simulink model "seMM1QueuingSys"  (R2024a)
settings: Solver=VariableStepAuto  StartTime=0.0  StopTime=60  RelTol=1e-3  EnableMultiTasking=on
model workspace (MAT data in the model file):
  GGwp = 5
undefined symbols (not defined in the file): m, n
libraries: commrandsrc3 x8, spsMonostableLib x4, simulink x2
settings Model: SimulationMode=accelerator  Creator=The MathWorks, Inc.  LastModifiedBy=94410
settings SolverCC: AlgebraicLoopSolver=TrustRegion
settings DataIOCC: LimitDataPoints=on  SaveFormat=Array  ReturnWorkspaceOutputs=off
settings OptimizationCC: LifeSpan=inf
settings DebuggingCC: UnconnectedInputMsg=warning  UnconnectedOutputMsg=warning  UnconnectedLineMsg=warning  AllowSymbolicDim=off  SFUnexpectedBacktrackingDiag=warning  SFNoUnconditionalDefaultTransitionDiag=warning  SFExecutionAtInitializationDiag=none  ArithmeticOperatorsInVariantConditions=warning
settings ModelReferenceCC: EnableRefExpFcnMdlSchedulingChecks=on  PropagateSignalLabelsOutOfModel=off
settings SFSimCC: SimUseLocalCustomCode=off  CustomCodeUndefinedFunction=UseInterfaceOnly
settings RTWCC: RTWUseLocalCustomCode=off  GPUComputeCapability=3.5  DLArmComputeVersion=19.05
settings CodeAppCC: StateflowObjectComments=on
settings GRTTargetCC: TargetLangStandard=C89/C90 (ANSI)
settings ConfigComp: CovMetricSettings=dw  CovSaveCumulativeToWorkspaceVar=on  CovSaveSingleToWorkspaceVar=on  CovExternalEMLEnable=off  CovSFcnEnable=off

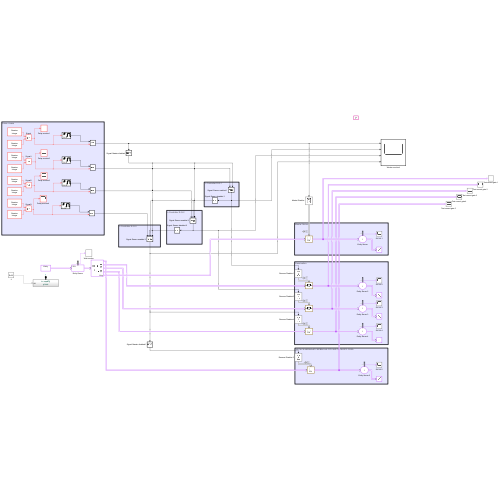
[thumbnail: Simulink's stored preview of the top-level diagram]
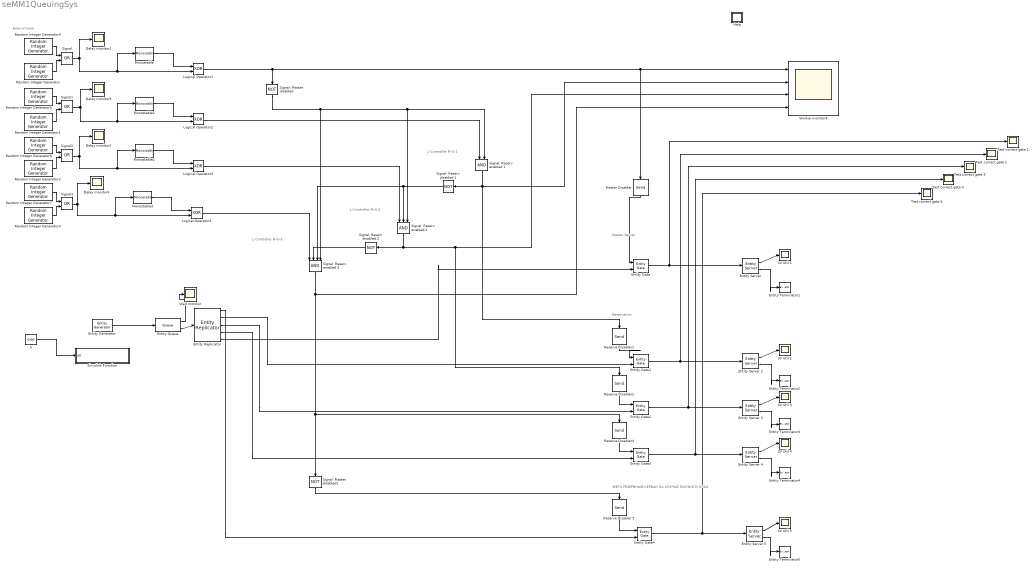
== system seMM1QueuingSys ==
  note: МЕГА РЕЗЕРВНЫЙ СЕРВАК НА СЛУЧАЙ ПОЛНОГО ОЧКА
  note: L-Controller R-G-3
  note: L-Controller R-G-2
  note: L-Controller R-G-1
  note: Reservation
  note: Master Server
  note: Блок отказа
  " λ" : Constant  Value=0.66  SampleTime=-1
  Delay monitor{1..4} (4 alike) : Scope
  Entity Gate{,1..4} (5 alike) : EntityGate  InputPortMessageModes=m,m  OutputPortMessageModes=m
  Entity Generator : EntityGenerator  OutputPortMessageModes=m  TimeSource=MATLAB action  Period=5  IntergenerationTimeAction=dt = expAT();  AttributeName=entity  AttributeInitialValue=0  EntityType=Structured  EntityTypeName=Entity
  Entity Queue : Queue  InputPortMessageModes=m  OutputPortMessageModes=n,m  Capacity=inf  AverageWait=on
      settings: OutputPortMap=o2,o5
  Entity Replicator : EntityReplicator  InputPortMessageModes=m  OutputPortMessageModes=m,m,m,m,m  NumberReplicas=4
      settings: OutputPortMap=o0,o1,o2,o3,o4
  Entity Server : EntityServer  InputPortMessageModes=m  OutputPortMessageModes=n,m  Capacity=1  ServiceTimeValue=2.0  Utilization=on
      settings: OutputPortMap=o5,o9
  Entity Server {2..5} (4 alike) : EntityServer  InputPortMessageModes=m  OutputPortMessageModes=n,m  Capacity=1  ServiceTimeValue=2.0  Utilization=on
      settings: OutputPortMap=o5,o9
  Entity Terminator{1..5} (5 alike) : EntityTerminator  InputPortMessageModes=m
  Help : Subsystem
      settings: OpenFcn=showExample('simevents/MM1QueuingSysExample');
      mask Display: disp('?')
  Logical Operator{1..4} (4 alike) : Logic  Operator=XOR  AllPortsSameDT=off  OutDataTypeStr=boolean
  Master Disabler : Send  OutputPortMessageModes=m
  Monostable{,1..3} (4 alike) : spsMonostableLib/Monostable  EdgeDetect=Rising  PulseDuration=0.5  ic=1  Ts=0
      settings: LibrarySourceBlock=sps_lib/Control/Monostable
  Random Integer Generator : commrandsrc3/Random Integer Generator  SetSize=2  SeedSource=Parameter  Seed=440  SampleTime=1  SamplesPerFrame=1  OutputDataType=boolean  SimulateUsing=Interpreted execution
  Random Integer Generator1 : commrandsrc3/Random Integer Generator  SetSize=2  SeedSource=Parameter  Seed=706  SampleTime=1  SamplesPerFrame=1  OutputDataType=boolean  SimulateUsing=Interpreted execution
  Random Integer Generator2 : commrandsrc3/Random Integer Generator  SetSize=2  SeedSource=Parameter  Seed=569  SampleTime=1  SamplesPerFrame=1  OutputDataType=boolean  SimulateUsing=Interpreted execution
  Random Integer Generator3 : commrandsrc3/Random Integer Generator  SetSize=2  SeedSource=Parameter  Seed=513  SampleTime=1  SamplesPerFrame=1  OutputDataType=boolean  SimulateUsing=Interpreted execution
  Random Integer Generator4 : commrandsrc3/Random Integer Generator  SetSize=2  SeedSource=Parameter  Seed=420  SampleTime=1  SamplesPerFrame=1  OutputDataType=boolean  SimulateUsing=Interpreted execution
  Random Integer Generator5 : commrandsrc3/Random Integer Generator  SetSize=2  SeedSource=Parameter  Seed=700  SampleTime=1  SamplesPerFrame=1  OutputDataType=boolean  SimulateUsing=Interpreted execution
  Random Integer Generator6 : commrandsrc3/Random Integer Generator  SetSize=2  SeedSource=Parameter  Seed=560  SampleTime=1  SamplesPerFrame=1  OutputDataType=boolean  SimulateUsing=Interpreted execution
  Random Integer Generator7 : commrandsrc3/Random Integer Generator  SetSize=2  SeedSource=Parameter  Seed=430  SampleTime=1  SamplesPerFrame=1  OutputDataType=boolean  SimulateUsing=Interpreted execution
  Reserve Disabler 5 : Send  OutputPortMessageModes=m
  Reserve Disabler1 : Send  OutputPortMessageModes=m
  Reserve Disabler2 : Send  OutputPortMessageModes=m
  Reserve Disabler4 : Send  OutputPortMessageModes=m
  SV Util {1..5} (5 alike) : Scope
  Signal{,1..3} (4 alike) : Logic  Operator=OR  AllPortsSameDT=off  OutDataTypeStr=boolean
  Signal: Master disabled : Logic  Operator=NOT  AllPortsSameDT=off  OutDataTypeStr=boolean
  Signal: Master disabled1 : Logic  Operator=NOT  AllPortsSameDT=off  OutDataTypeStr=boolean
  Signal: Reserv disabled 1 : Logic  Operator=NOT  AllPortsSameDT=off  OutDataTypeStr=boolean
  Signal: Reserv disabled 2 : Logic  Operator=NOT  AllPortsSameDT=off  OutDataTypeStr=boolean
  Signal: Reserv enabled 1 : Logic  AllPortsSameDT=off  OutDataTypeStr=boolean
  Signal: Reserv enabled 2 : Logic  Inputs=3  AllPortsSameDT=off  OutDataTypeStr=boolean
  Signal: Reserv enabled 3 : Logic  Inputs=4  AllPortsSameDT=off  OutDataTypeStr=boolean
  Simulink Function : Subsystem  TreatAsAtomicUnit=on
  Test correct gate {1..5} (5 alike) : Scope
  Wait monitor : Scope
  Worker monitor4 : Scope  NumInputPorts=4
  wires:
  " λ"/1 -> Simulink Function/1(AR)
  Entity Gate/1 -> Entity Server/1, Test correct gate 1/1
  Entity Generator/1 -> Entity Queue/1
  Entity Gate1/1 -> Entity Server 2/1, Test correct gate 2/1
  Entity Queue/2 -> Entity Replicator/1
  Entity Queue/1 -> Wait monitor/1
  Entity Replicator/1 -> Entity Gate4/2
  Entity Replicator/2 -> Entity Gate1/2
  Entity Server/2 -> Entity Terminator1/1
  Entity Server 2/2 -> Entity Terminator2/1
  Signal/1 -> Delay monitor1/1, Monostable/1, Logical Operator1/2
  Entity Server/1 -> SV Util 1/1
  Entity Server 2/1 -> SV Util 2/1
  Monostable/1 -> Logical Operator1/1
  Monostable1/1 -> Logical Operator2/1
  Signal1/1 -> Delay monitor3/1, Monostable1/1, Logical Operator2/2
  Entity Server 3/1 -> SV Util 3/1
  Entity Server 4/1 -> SV Util 4/1
  Entity Server 4/2 -> Entity Terminator4/1
  Entity Server 3/2 -> Entity Terminator3/1
  Entity Replicator/3 -> Entity Gate2/2
  Entity Replicator/4 -> Entity Gate3/2
  Entity Gate2/1 -> Entity Server 3/1, Test correct gate 3/1
  Entity Gate3/1 -> Entity Server 4/1, Test correct gate 4/1
  Master Disabler/1 -> Entity Gate/1
  Logical Operator1/1 -> Master Disabler/1, Worker monitor4/1, Signal: Master disabled/1
  Reserve Disabler1/1 -> Entity Gate1/1
  Reserve Disabler2/1 -> Entity Gate2/1
  Reserve Disabler4/1 -> Entity Gate3/1
  Signal: Master disabled/1 -> Signal: Reserv enabled 3/4, Signal: Reserv enabled 2/3, Signal: Reserv enabled 1/2
  Logical Operator2/1 -> Signal: Reserv enabled 1/1
  Signal: Reserv enabled 1/1 -> Worker monitor4/2, Signal: Reserv disabled 1/1, Reserve Disabler1/1
  Signal2/1 -> Monostable2/1, Logical Operator3/2, Delay monitor2/1
  Monostable2/1 -> Logical Operator3/1
  Signal3/1 -> Delay monitor4/1, Monostable3/1, Logical Operator4/2
  Monostable3/1 -> Logical Operator4/1
  Signal: Reserv disabled 1/1 -> Signal: Reserv enabled 3/3, Signal: Reserv enabled 2/2
  Logical Operator3/1 -> Signal: Reserv enabled 2/1
  Signal: Reserv enabled 2/1 -> Worker monitor4/3, Reserve Disabler2/1, Signal: Reserv disabled 2/1
  Signal: Reserv disabled 2/1 -> Signal: Reserv enabled 3/2
  Logical Operator4/1 -> Signal: Reserv enabled 3/1
  Signal: Reserv enabled 3/1 -> Worker monitor4/4, Signal: Master disabled1/1, Reserve Disabler4/1
  Entity Gate4/1 -> Entity Server 5/1, Test correct gate 5/1
  Entity Server 5/1 -> SV Util 5/1
  Entity Server 5/2 -> Entity Terminator5/1
  Signal: Master disabled1/1 -> Reserve Disabler 5/1
  Entity Replicator/5 -> Entity Gate/2
  Reserve Disabler 5/1 -> Entity Gate4/1
  Random Integer Generator4/1 -> Signal/1
  Random Integer Generator/1 -> Signal/2
  Random Integer Generator5/1 -> Signal1/1
  Random Integer Generator1/1 -> Signal1/2
  Random Integer Generator6/1 -> Signal2/1
  Random Integer Generator2/1 -> Signal2/2
  Random Integer Generator7/1 -> Signal3/1
  Random Integer Generator3/1 -> Signal3/2

== system seMM1QueuingSys/Help ==

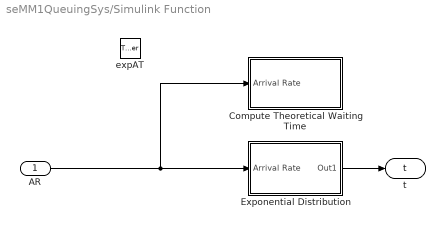
== system seMM1QueuingSys/Simulink Function ==
  AR : Inport
  expAT : TriggerPort  TriggerType=function-call  IsSimulinkFunction=on  FunctionName=expAT  VariantControl=Variant
  Compute Theoretical Waiting Time : Subsystem
  Exponential Distribution : Subsystem
  t : ArgOut  DisableCoverage=on  ArgumentName=t
  wires:
  AR/1 -> Compute Theoretical Waiting Time/1(Arrival Rate), Exponential Distribution/1(Arrival Rate)
  Exponential Distribution/1(Out1) -> t/1

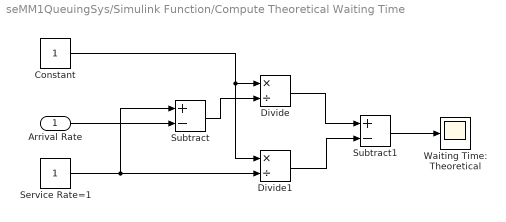
== system seMM1QueuingSys/Simulink Function/Compute Theoretical Waiting Time ==
  Arrival Rate : Inport
  Constant : Constant
  Divide : Product  Inputs=*/
  Divide1 : Product  Inputs=*/
  Service Rate=1 : Constant
  Subtract : Sum  Inputs=+-
  Subtract1 : Sum  Inputs=+-
  Waiting Time: Theoretical : Scope
  wires:
  Arrival Rate/1 -> Subtract/2
  Subtract1/1 -> Waiting Time: Theoretical/1
  Divide1/1 -> Subtract1/2
  Divide/1 -> Subtract1/1
  Subtract/1 -> Divide/2
  Constant/1 -> Divide1/1, Divide/1
  Service Rate=1/1 -> Subtract/1, Divide1/2

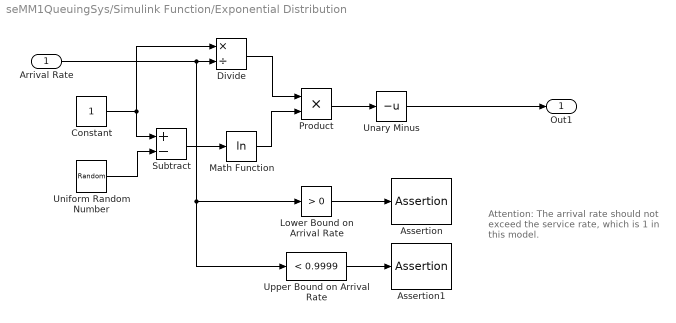
== system seMM1QueuingSys/Simulink Function/Exponential Distribution ==
  note: Attention: The arrival rate
      | should not exceed the service
      | rate, which is 1 in this model.
  Arrival Rate : Inport
  Assertion : Assertion
  Assertion1 : Assertion
  Constant : Constant
  Divide : Product  Inputs=*/
  Lower Bound on Arrival Rate : simulink/Logic and Bit Operations/Compare To Constant  relop=>  const=0  OutDataTypeStr=uint8  ZeroCross=off
  Math Function : Math  Operator=log  SignedPower=on
  Product : Product  RndMeth=Zero
  Subtract : Sum  Inputs=+-
  Unary Minus : UnaryMinus
  Uniform Random Number : UniformRandomNumber  Minimum=0  Seed=12345
  "Upper Bound on Arrival Rate " : simulink/Logic and Bit Operations/Compare To Constant  relop=<  const=0.9999  OutDataTypeStr=uint8  ZeroCross=off
  Out1 : Outport
  wires:
  Arrival Rate/1 -> Divide/2, Lower Bound on Arrival Rate/1, "Upper Bound on Arrival Rate "/1
  Unary Minus/1 -> Out1/1
  Product/1 -> Unary Minus/1
  Math Function/1 -> Product/2
  Divide/1 -> Product/1
  Constant/1 -> Divide/1, Subtract/1
  Uniform Random Number/1 -> Subtract/2
  Lower Bound on Arrival Rate/1 -> Assertion/1
  "Upper Bound on Arrival Rate "/1 -> Assertion1/1
  Subtract/1 -> Math Function/1
